simulink model "motor_position_ctrl"  (R2020a)
settings: Solver=VariableStepAuto  StartTime=0.0  StopTime=10.0  RelTol=1e-3
undefined symbols (not defined in the file or in its folder): b, J, K, L, R
settings Model: Creator=Shubham  LastModifiedBy=Shubham

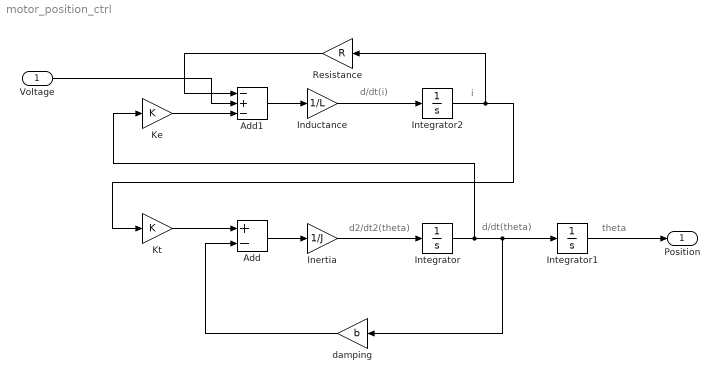
== system motor_position_ctrl ==
  note: d/dt(i)
  note: d/dt(theta)
  note: theta
  note: d2/dt2(theta)
  note: i
  Voltage : Inport
  Add : Sum  Inputs=+-
  Add1 : Sum  Inputs=-+-
  Inductance : Gain  Gain=1/L
  Inertia : Gain  Gain=1/J
  Integrator : Integrator
  Integrator1 : Integrator
  Integrator2 : Integrator
  Ke : Gain  Gain=K
  Kt : Gain  Gain=K
  Resistance : Gain  Gain=R
  damping : Gain  Gain=b
  Position : Outport
  wires:
  Resistance/1 -> Add1/1
  Kt/1 -> Add/1
  Integrator1/1 -> Position/1
  Add/1 -> Inertia/1
  damping/1 -> Add/2
  Ke/1 -> Add1/3
  Add1/1 -> Inductance/1
  Voltage/1 -> Add1/2
  Inertia/1 -> Integrator/1
  Integrator/1 -> Ke/1, damping/1, Integrator1/1
  Integrator2/1 -> Resistance/1, Kt/1
  Inductance/1 -> Integrator2/1
